simulink model "step_4_r2021a"  (R2021a)
settings: Solver=VariableStepAuto  StartTime=0.0  StopTime=0.2  RelTol=1e-3
undefined symbols (not defined in the file): bm, Jm, Kt, L, R
libraries: fl_lib x12, nesl_utility x3, ee_lib x1, sdl_lib x1
settings Model: Creator=mfussi  LastModifiedBy=mfussi

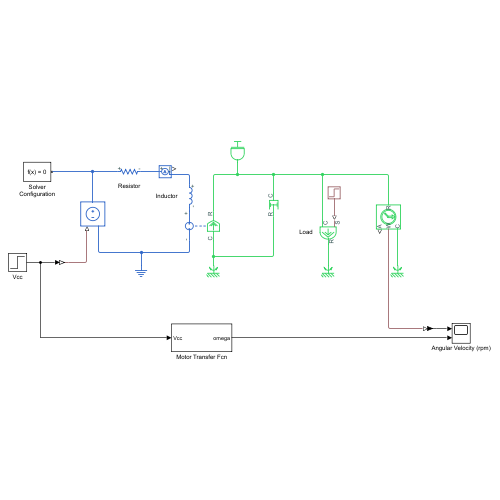
[thumbnail: Simulink's stored preview of the top-level diagram]
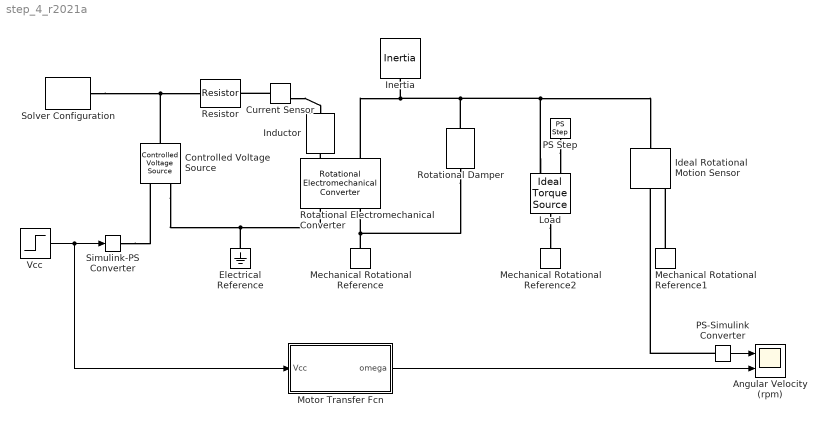
== system step_4_r2021a ==
  Angular Velocity (rpm) : Scope  NumInputPorts=2
  Controlled Voltage Source : fl_lib/Electrical/Electrical Sources/Controlled Voltage Source
  Current Sensor : fl_lib/Electrical/Electrical Sensors/Current Sensor
  Electrical Reference : fl_lib/Electrical/Electrical Elements/Electrical Reference
  Ideal Rotational Motion Sensor : fl_lib/Mechanical/Mechanical Sensors/Ideal Rotational Motion Sensor  wrap_angle=simscape.enum.onoff.off  offset=0 rad
  Inductor : ee_lib/Passive/Inductor  l=L uH  L_tol=0  enable_L_tol=0  tol_distribution=1  nSigma=4  r=0 Ohm  g=0 1/Ohm  enable_operating_limits=0  operating_limit_action=2  max_working_current=1 A  power_rating=1 W  enable_faults=0  fault_action=1  lambdaPercent=50  k_faulted=0.9999  turnsShort=0  openCct=0  groundShort=0  groundShortG=0 1/Ohm  tau_fault=1e-3 s  enable_temporal_fault=0  t_fault=1 s  enable_behavioral_fault=0  max_permissible_voltage=100 V  n_fail_on_voltage=1  max_permissible_current=1 A  t_fail_on_current=1 s  i_L_specify=off  i_L_priority=High  i_L=0 A  i_L_nominal_specify=off  i_L_nominal_unit=A  i_L_nominal_value=1
  Inertia : fl_lib/Mechanical/Rotational Elements/Inertia  inertia=Jm g*cm^2  num_ports=foundation.enum.numPorts2.one  w_specify=off  w_priority=High  w=0 rad/s  w_nominal_specify=off  w_nominal_unit=rad/s  w_nominal_value=1  t_specify=off  t_priority=None  t=0 N*m  t_nominal_specify=off  t_nominal_unit=N*m  t_nominal_value=1
  Load : fl_lib/Mechanical/Mechanical Sources/Ideal Torque Source
  Mechanical Rotational Reference : fl_lib/Mechanical/Rotational Elements/Mechanical Rotational Reference
  Mechanical Rotational Reference1 : fl_lib/Mechanical/Rotational Elements/Mechanical Rotational Reference
  Mechanical Rotational Reference2 : fl_lib/Mechanical/Rotational Elements/Mechanical Rotational Reference
  Motor Transfer Fcn : Subsystem
  PS Step : fl_lib/Physical Signals/Sources/PS Step  step_time=0.1 s  initial_value=0  final_value=0.01 N*m
      settings: SourceProductBaseCode=SS
  PS-Simulink Converter : nesl_utility/PS-Simulink Converter  PhysicalDomain=network_engine_domain  SubClassName=ps_output  LeftPortType=input  RightPortType=output  PseudoPeriodic=off  Frequencies=[]  Unit=rpm  AffineConversion=off
      settings: SourceProductBaseCode=PW,SS
  Resistor : fl_lib/Electrical/Electrical Elements/Resistor  R=R Ohm  i_specify=off  i_priority=None  i=0 A  i_nominal_specify=off  i_nominal_unit=A  i_nominal_value=1  v_specify=off  v_priority=None  v=0 V  v_nominal_specify=off  v_nominal_unit=V  v_nominal_value=1
  Rotational Electromechanical Converter : fl_lib/Electrical/Electrical Elements/Rotational Electromechanical Converter  K=Kt mN*m/A  i_specify=off  i_priority=None  i=0 A  i_nominal_specify=off  i_nominal_unit=A  i_nominal_value=1  v_specify=off  v_priority=None  v=0 V  v_nominal_specify=off  v_nominal_unit=V  v_nominal_value=1  t_specify=off  t_priority=None  t=0 N*m  t_nominal_specify=off  t_nominal_unit=N*m  t_nominal_value=1  w_specify=off  w_priority=None  w=0 rad/s  w_nominal_specify=off  w_nominal_unit=rad/s  w_nominal_value=1
  Rotational Damper : sdl_lib/Couplings & Drives/Springs & Dampers/Rotational Damper  D=bm m*mN/rpm  enable_faults=simscape.enum.onoff.off  b_fault=100 N*m/(rad/s)  temporal_fault=simscape.enum.onoff.off  fault_time=5 s  shock_fault=simscape.enum.onoff.off  acceleration_limit=100 rad/s^2  shock_limit=1  report_fault=simscape.enum.assert.action.none  thermal_port=simscape.enum.thermaleffects.omit  thermal_mass=50 kJ/K  temperature_specify=off  temperature_priority=High  temperature=300 K  temperature_nominal_specify=off  temperature_nominal_unit=K  temperature_nominal_value=1
      settings: SourceProductBaseCode=LD
  Simulink-PS Converter : nesl_utility/Simulink-PS Converter  PhysicalDomain=network_engine_domain  SubClassName=ps_input  LeftPortType=input  RightPortType=output  PseudoPeriodic=off  Frequencies=[]  NoiseDistribution=none  NoiseParameters=[]  Unit=1  AffineConversion=off  FilteringAndDerivatives=provide  SimscapeFilterOrder=1  InputFilterTimeConstant=0.001  UdotUserProvided=0
      settings: SourceProductBaseCode=PW,SS
  Solver Configuration : nesl_utility/Solver Configuration  PhysicalDomain=network_engine_domain  SubClassName=solver  LeftPortType=input  RightPortType=generic  Tones=[]  Harmonics=[]  SimulateNoise=off  Profile=off  UseLocalSampling=off  EnableSwitchedLinearOptims=on  FrequencyDomain=off  UseCCode=off  RelTol=0.001  AbsTol=1e-06  MinStep=1e-09  ToWorkspace=off  RevertToSquareIcSolve=off  NumHomotopyIterations=100  PhasorMode=off  PhasorModeNumHarmonics=1  DoDC=off  ResidualTolerance=1e-09  UseLocalSolver=off  LocalSolverChoice=NE_BACKWARD_EULER_ADVANCER  LocalSolverSampleTime=0.001  DoFixedCost=off  MaxNonlinIter=3  MaxModeIter=2  ComputeImpulses=off  ImpulseIterations=2  LinearAlgebra=auto  EquationFormulation=NE_TIME_EF  DelaysMemoryBudget=1024  AutomaticFiltering=on  FilteringTimeConstant=0.001  PartitionStorageMethod=AS_NEEDED  PartitionMemoryBudget=1024  PartitionMethod=ROBUST
      settings: SourceProductBaseCode=PW,SS
  Vcc : Step  Time=1e-4  SampleTime=0
  wires:
  Vcc/1 -> Motor Transfer Fcn/1(Vcc), Simulink-PS Converter/1
  Motor Transfer Fcn/1(omega) -> Angular Velocity (rpm)/2
  PS-Simulink Converter/1 -> Angular Velocity (rpm)/1
  connections:
  Current Sensor/LConn1 -- Resistor/RConn1
  Controlled Voltage Source/LConn1 -- Resistor/LConn1 -- Solver Configuration/RConn1
  Simulink-PS Converter/RConn1 -- Controlled Voltage Source/RConn1
  Rotational Electromechanical Converter/LConn1 -- Inductor/RConn1
  Controlled Voltage Source/RConn2 -- Rotational Electromechanical Converter/RConn1 -- Electrical Reference/LConn1
  Mechanical Rotational Reference/LConn1 -- Rotational Damper/LConn1 -- Rotational Electromechanical Converter/RConn2
  Load/RConn2 -- Ideal Rotational Motion Sensor/LConn1 -- Rotational Damper/RConn1 -- Rotational Electromechanical Converter/LConn2 -- Inertia/LConn1
  Current Sensor/RConn2 -- Inductor/LConn1
  PS-Simulink Converter/LConn1 -- Ideal Rotational Motion Sensor/RConn2
  Mechanical Rotational Reference1/LConn1 -- Ideal Rotational Motion Sensor/RConn1
  Load/LConn1 -- Mechanical Rotational Reference2/LConn1
  PS Step/RConn1 -- Load/RConn1

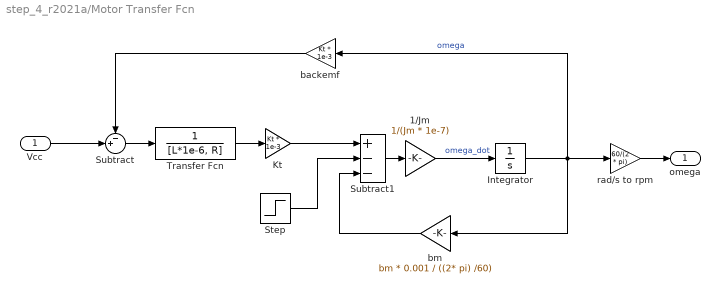
== system step_4_r2021a/Motor Transfer Fcn ==
  Vcc : Inport
  1/Jm : Gain  Gain=1/(Jm * 1e-7)
  Integrator : Integrator  ContinuousStateAttributes='omega'
  Kt : Gain  Gain=Kt * 1e-3
  Step : Step  Time=0.1  After=0.01  SampleTime=0
  Subtract : Sum  Inputs=-+|
  Subtract1 : Sum  Inputs=+--
  Transfer Fcn : TransferFcn  Denominator=[L*1e-6, R]
  backemf : Gain  Gain=Kt * 1e-3
  bm : Gain  Gain=bm * 0.001 / ((2* pi) /60)
  rad/s to rpm : Gain  Gain=60/(2 * pi)
  omega : Outport
  wires:
  Vcc/1 -> Subtract/2
  Transfer Fcn/1 -> Kt/1
  Integrator/1 -> bm/1, rad/s to rpm/1, backemf/1  "omega"
  backemf/1 -> Subtract/1
  1/Jm/1 -> Integrator/1  "omega_dot"
  Subtract/1 -> Transfer Fcn/1
  rad/s to rpm/1 -> omega/1
  Kt/1 -> Subtract1/1
  Subtract1/1 -> 1/Jm/1
  bm/1 -> Subtract1/3
  Step/1 -> Subtract1/2
